simulink model "mass_damper_spring_custom_plant"  (R2015b)
settings: Solver=VariableStepAuto  StartTime=0.0  StopTime=100  RelTol=1e-3
settings Model: Creator=galey  LastModifiedBy=galey

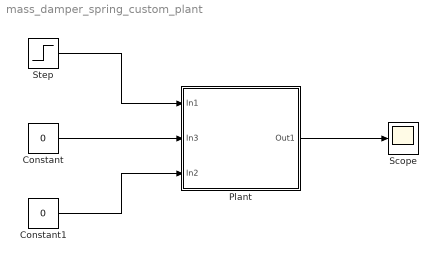
== system mass_damper_spring_custom_plant ==
  Constant : Constant  Value=0
  Constant1 : Constant  Value=0
  Plant : Subsystem
  Scope : Scope
  Step : Step  Time=50  SampleTime=0
  wires:
  Plant/1(Out1) -> Scope/1
  Constant/1 -> Plant/2(In3)
  Constant1/1 -> Plant/3(In2)
  Step/1 -> Plant/1(In1)

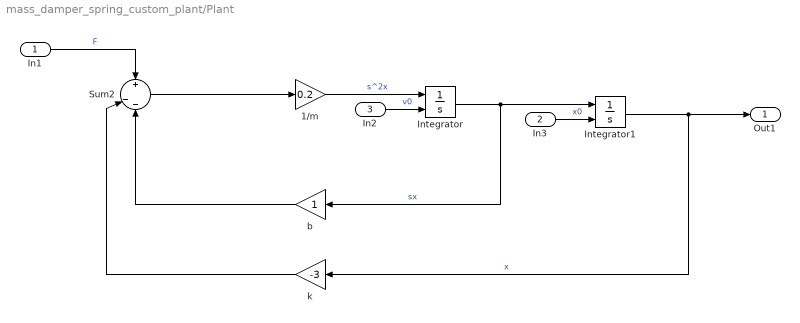
== system mass_damper_spring_custom_plant/Plant ==
  In1 : Inport
  In3 : Inport  Port=2
  In2 : Inport  Port=3
  1/m : Gain  Gain=0.2
  Integrator : Integrator  InitialConditionSource=external
  Integrator1 : Integrator  InitialConditionSource=external
  Sum2 : Sum  Inputs=+|--
  b : Gain
  k : Gain  Gain=-3
  Out1 : Outport
  wires:
  Integrator/1 -> b/1, Integrator1/1  "sx"
  Integrator1/1 -> Out1/1, k/1  "x"
  b/1 -> Sum2/3
  In1/1 -> Sum2/1  "F"
  In2/1 -> Integrator/2  "v0"
  Sum2/1 -> 1/m/1
  1/m/1 -> Integrator/1  "s^2x"
  k/1 -> Sum2/2
  In3/1 -> Integrator1/2  "x0"
